simulink model "slave_task"  (Simulink 7.1)
libraries: mathlib x12
settings Model: Creator=jsobota  LastModifiedBy=jsobota  ExtModeTrigMode=oneshot  ExtModeArmWhenConnect=off

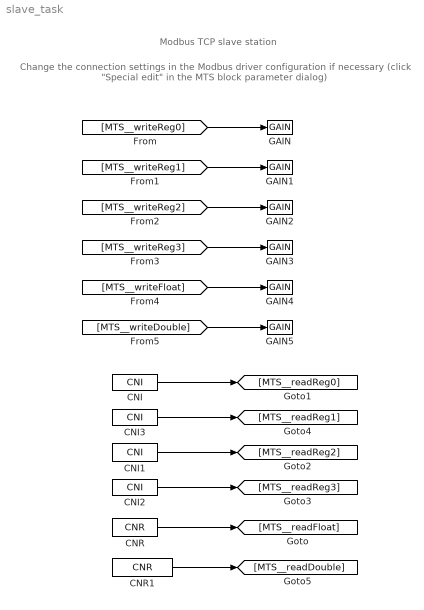
== system slave_task ==
  note: Modbus TCP slave station
  note: Change the connection settings in the Modbus driver configuration
      | if necessary (click "Special edit" in the MTS block parameter dialog)
  CNI : mathlib/CNI  icn=91
  CNI1 : mathlib/CNI  icn=65432
  CNI2 : mathlib/CNI  icn=-32132
  CNI3 : mathlib/CNI  icn=-76
  CNR : mathlib/CNR  ycn=-32.76
  CNR1 : mathlib/CNR  ycn=-98765.2
  GAIN{,1..5} (6 alike) : mathlib/GAIN  k=1
  wires:
  CNI/1 -> [MTS__readReg0]
  CNI1/1 -> [MTS__readReg2]
  CNI2/1 -> [MTS__readReg3]
  CNI3/1 -> [MTS__readReg1]
  CNR/1 -> [MTS__readFloat]
  CNR1/1 -> [MTS__readDouble]
  [MTS__writeReg0] -> GAIN/1
  [MTS__writeReg1] -> GAIN1/1
  [MTS__writeReg2] -> GAIN2/1
  [MTS__writeReg3] -> GAIN3/1
  [MTS__writeFloat] -> GAIN4/1
  [MTS__writeDouble] -> GAIN5/1
